simulink model "Model"  (R2018b)
settings: Solver=VariableStepAuto  StartTime=0.0  StopTime=20  MaxStep=0.001  RelTol=1e-3
libraries: fl_lib x12, nesl_utility x9, sh_lib x5
settings Model: Creator=admin  LastModifiedBy=Ervin
settings SolverCC: MaxConsecutiveMinStep=5  AlgebraicLoopSolver=LineSearch
settings DebuggingCC: LibraryContextMissingDiagnostic=none
settings SFSimCC: SimUseLocalCustomCode=off
settings RTWCC: RTWUseLocalCustomCode=off
settings SimscapeCC: SimscapeLogType=all  SimscapeLogDataHistory=100000000

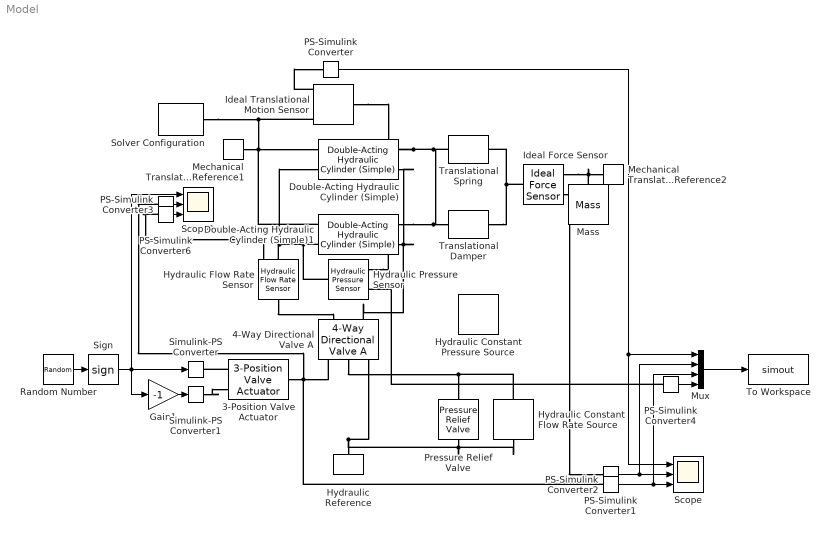
== system Model ==
  3-Position Valve Actuator : sh_lib/Valves/Valve Actuators/3-Position Valve Actuator  stroke=0.005 m  t_on=0.15 s  t_off=0.15 s  act_signal=1  init_position=2
      settings: SourceProductName=Simscape Fluids  SourceProductBaseCode=SH
  4-Way Directional Valve A : sh_lib/Valves/Directional Valves/4-Way Directional Valve A  mdl_type=1  area_max=0.5e-4 m^2  opening_max=0.005 m  opening_tab=[-.002, 0, .002, .005, .015] m  area_tab=[1e-09, 2.0352e-07, 4.0736e-05, .00011438, .00034356] m^2  pressure_tab=[-10000000, -5000000, -2000000, 2000000, 5000000, 10000000] Pa  flow_rate_tab=[-1e-07, -7.0711e-08, -4.4721e-08, 4.4721e-08, 7.0711e-08, 1e-07; -2.0352e-05, -1.4391e-05, -9.1017e-06, 9.1017e-06, 1.4391e-05, 2.0352e-05; -.0040736, -.0028805, -.0018218, .0018218, .0028805, .0040736; -.011438, -.0080879, -.0051152, .0051152, .0080879, .011438; -.034356, -.024293, -.015364, .015364, .024293, .034356] m^3/s  interp_method=1  extrap_method=1  C_d=0.7  x_0_P_A=-2.5e-3 m  x_0_P_B=-2.5e-3 m  x_0_A_T=-2.5e-3 m  x_0_B_T=-2.5e-3 m  x_0_P_T1=2.5e-3 m  x_0_T1_T=2.5e-3 m  A_leak=1e-12 m^2  lam_spec=1  B_lam=0.999  Re_cr=12
      settings: SourceProductName=Simscape Fluids  SourceProductBaseCode=SH  LogSimulationData=on
  Double-Acting Hydraulic Cylinder (Simple) : sh_lib/Hydraulic Cylinders/Double-Acting Hydraulic Cylinder (Simple)  area_A=49*pi/4 cm^2  area_B=(49-25)*pi/4 cm^2  stroke=72 cm  init_pos=0 cm  penetr_coeff=1e20 s*N/m^2  or=1
      settings: SourceProductName=Simscape Fluids  SourceProductBaseCode=SH
  Double-Acting Hydraulic Cylinder (Simple)1 : sh_lib/Hydraulic Cylinders/Double-Acting Hydraulic Cylinder (Simple)  area_A=49*pi/4 cm^2  area_B=(49-25)*pi/4 cm^2  stroke=72 cm  init_pos=0 cm  penetr_coeff=1e20 s*N/m^2  or=1
      settings: SourceProductName=Simscape Fluids  SourceProductBaseCode=SH
  Gain1 : Gain  Gain=-1
  Hydraulic Constant Flow Rate Source : fl_lib/Hydraulic/Hydraulic Sources/Hydraulic Constant Flow Rate Source  commanded_flow_rate=0.3 m^3/s
      settings: SourceProductName=Simscape  SourceProductBaseCode=SS
  Hydraulic Constant Pressure Source : fl_lib/Hydraulic/Hydraulic Sources/Hydraulic Constant Pressure Source  commanded_pressure=5e7 Pa
      settings: SourceProductName=Simscape  SourceProductBaseCode=SS
  Hydraulic Flow Rate Sensor : fl_lib/Hydraulic/Hydraulic Sensors/Hydraulic Flow Rate Sensor
      settings: SourceProductName=Simscape
  Hydraulic Pressure Sensor : fl_lib/Hydraulic/Hydraulic Sensors/Hydraulic Pressure Sensor
      settings: SourceProductName=Simscape
  Hydraulic Reference : fl_lib/Hydraulic/Hydraulic Elements/Hydraulic Reference
      settings: SourceProductName=Simscape
  Ideal Force Sensor : fl_lib/Mechanical/Mechanical Sensors/Ideal Force Sensor
  Ideal Translational Motion Sensor : fl_lib/Mechanical/Mechanical Sensors/Ideal Translational Motion Sensor  offset=0 m
  Mass : fl_lib/Mechanical/Translational Elements/Mass  mass=180 kg  v_specify=off  v_priority=High  v=0 m/s  v_nominal_specify=off  v_nominal_unit=m/s  v_nominal_value=1  f_specify=off  f_priority=None  f=0 N  f_nominal_specify=off  f_nominal_unit=N  f_nominal_value=1
  Mechanical Translational Reference1 : fl_lib/Mechanical/Translational Elements/Mechanical Translational Reference
  Mechanical Translational Reference2 : fl_lib/Mechanical/Translational Elements/Mechanical Translational Reference
  Mux : Mux
  PS-Simulink Converter{,1..4,6} (6 alike) : nesl_utility/PS-Simulink Converter  PhysicalDomain=network_engine_domain  SubClassName=ps_output  LeftPortType=input  RightPortType=output  PseudoPeriodic=off  Frequencies=[]  Unit=1  AffineConversion=off
  Pressure Relief Valve : sh_lib/Valves/Pressure Control Valves/Pressure Relief Valve  valve_area_spec=1  p_diff_TLU=[30.15e5 : 15e3 : 31.35e5] Pa  area_TLU=[1 : 1 : 9] .* 1e-5 m^2  area_max=0.001 m^2  pres_set=1e7 Pa  reg_range=1e7 Pa  C_d=0.7  A_leak=1e-12 m^2  lam_spec=1  B_lam=0.999  Re_cr=12  dynamic=0  tau=0.1 s  area_init=1e-12 m^2
      settings: SourceProductName=Simscape Fluids  SourceProductBaseCode=SH
  Random Number : RandomNumber  Seed=18  SampleTime=2
  Scope : Scope  NumInputPorts=3
  Scope1 : Scope  NumInputPorts=3
  Sign : Signum
  Simulink-PS Converter : nesl_utility/Simulink-PS Converter  PhysicalDomain=network_engine_domain  SubClassName=ps_input  LeftPortType=input  RightPortType=output  PseudoPeriodic=off  Frequencies=[]  NoiseDistribution=none  NoiseParameters=[]  Unit=1  AffineConversion=off  FilteringAndDerivatives=filter  SimscapeFilterOrder=1  InputFilterTimeConstant=0.001  UdotUserProvided=0
  Simulink-PS Converter1 : nesl_utility/Simulink-PS Converter  PhysicalDomain=network_engine_domain  SubClassName=ps_input  LeftPortType=input  RightPortType=output  PseudoPeriodic=off  Frequencies=[]  NoiseDistribution=none  NoiseParameters=[]  Unit=1  AffineConversion=off  FilteringAndDerivatives=filter  SimscapeFilterOrder=1  InputFilterTimeConstant=0.001  UdotUserProvided=0
  Solver Configuration : nesl_utility/Solver Configuration  PhysicalDomain=network_engine_domain  SubClassName=solver  LeftPortType=input  RightPortType=generic  Tones=[]  Harmonics=[]  SimulateNoise=off  Profile=off  UseLocalSampling=off  EnableSwitchedLinearOptims=on  FrequencyDomain=off  UseCCode=off  RelTol=0.001  AbsTol=1e-06  MinStep=1e-09  ToWorkspace=off  RevertToSquareIcSolve=off  NumHomotopyIterations=100  PhasorMode=off  PhasorModeNumHarmonics=1  DoDC=on  ResidualTolerance=1e-05  UseLocalSolver=off  LocalSolverChoice=NE_BACKWARD_EULER_ADVANCER  LocalSolverSampleTime=0.001  DoFixedCost=off  MaxNonlinIter=3  MaxModeIter=2  LinearAlgebra=auto  EquationFormulation=NE_TIME_EF  DelaysMemoryBudget=1024  AutomaticFiltering=on  FilteringTimeConstant=0.001  PartitionStorageMethod=AS_NEEDED  PartitionMemoryBudget=1024
  To Workspace : ToWorkspace  VariableName=simout  SaveFormat=Structure With Time  SampleTime=-1
  Translational Damper : fl_lib/Mechanical/Translational Elements/Translational Damper  D=400 N/(m/s)  v_specify=off  v_priority=None  v=0 m/s  v_nominal_specify=off  v_nominal_unit=m/s  v_nominal_value=1  f_specify=off  f_priority=None  f=0 N  f_nominal_specify=off  f_nominal_unit=N  f_nominal_value=1
  Translational Spring : fl_lib/Mechanical/Translational Elements/Translational Spring  spr_rate=40000 N/m  v_specify=off  v_priority=None  v=0 m/s  v_nominal_specify=off  v_nominal_unit=m/s  v_nominal_value=1  f_specify=off  f_priority=None  f=0 N  f_nominal_specify=off  f_nominal_unit=N  f_nominal_value=1  x_specify=off  x_priority=High  x=0 m  x_nominal_specify=off  x_nominal_unit=m  x_nominal_value=1
  wires:
  Random Number/1 -> Sign/1
  Sign/1 -> Gain1/1, Scope1/1, Simulink-PS Converter/1
  PS-Simulink Converter1/1 -> Mux/2, Scope/2
  Gain1/1 -> Simulink-PS Converter1/1
  PS-Simulink Converter6/1 -> Scope1/3
  PS-Simulink Converter/1 -> Scope/1, Mux/1
  PS-Simulink Converter2/1 -> Mux/3, Scope/3
  PS-Simulink Converter3/1 -> Scope1/2
  Mux/1 -> To Workspace/1
  PS-Simulink Converter4/1 -> Mux/4
  connections:
  Double-Acting Hydraulic Cylinder (Simple)1/LConn2 -- Hydraulic Pressure Sensor/LConn1 -- Hydraulic Flow Rate Sensor/RConn2 -- Double-Acting Hydraulic Cylinder (Simple)/LConn2
  Translational Damper/RConn1 -- Translational Spring/RConn1 -- Ideal Force Sensor/LConn1
  Double-Acting Hydraulic Cylinder (Simple)/RConn2 -- Hydraulic Pressure Sensor/RConn1 -- Double-Acting Hydraulic Cylinder (Simple)1/RConn2 -- 4-Way Directional Valve A/LConn2
  Mechanical Translational Reference1/LConn1 -- Solver Configuration/RConn1 -- Ideal Translational Motion Sensor/RConn1 -- Double-Acting Hydraulic Cylinder (Simple)1/LConn1 -- Double-Acting Hydraulic Cylinder (Simple)/LConn1
  Ideal Translational Motion Sensor/RConn3 -- PS-Simulink Converter/LConn1
  Mass/LConn1 -- Ideal Force Sensor/RConn1 -- Mechanical Translational Reference2/LConn1
  3-Position Valve Actuator/LConn1 -- Simulink-PS Converter/RConn1
  Translational Spring/LConn1 -- Double-Acting Hydraulic Cylinder (Simple)1/RConn1 -- Translational Damper/LConn1 -- Ideal Translational Motion Sensor/LConn1 -- Double-Acting Hydraulic Cylinder (Simple)/RConn1
  Simulink-PS Converter1/RConn1 -- 3-Position Valve Actuator/LConn2
  PS-Simulink Converter6/LConn1 -- Hydraulic Flow Rate Sensor/RConn1
  Hydraulic Flow Rate Sensor/LConn1 -- 4-Way Directional Valve A/LConn1
  3-Position Valve Actuator/RConn1 -- PS-Simulink Converter2/LConn1 -- PS-Simulink Converter3/LConn1 -- 4-Way Directional Valve A/RConn1
  Ideal Force Sensor/RConn2 -- PS-Simulink Converter1/LConn1
  4-Way Directional Valve A/RConn3 -- Pressure Relief Valve/RConn1 -- Hydraulic Constant Flow Rate Source/RConn1 -- Hydraulic Reference/LConn1
  4-Way Directional Valve A/RConn2 -- Hydraulic Constant Flow Rate Source/LConn1 -- Pressure Relief Valve/LConn1
  PS-Simulink Converter4/LConn1 -- Hydraulic Pressure Sensor/RConn2
